simulink model "linearPathDomainPlnt_th"  (R2018a)
settings: Solver=FixedStepAuto  StartTime=0.0  StopTime=simulationDuration_s  FixedStep=simulationTimeStep_s  RelTol=1e-3
libraries: linearPathDomainPlnt_cl x1
settings Model: Creator=mcobb  LastModifiedBy=mcobb

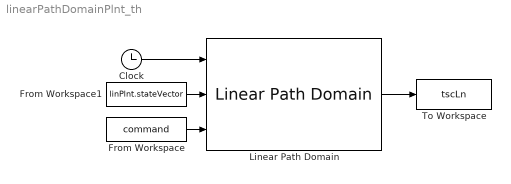
== system linearPathDomainPlnt_th ==
  Clock : Clock
  From Workspace : FromWorkspace  VariableName=command  SampleTime=0
  From Workspace1 : FromWorkspace  VariableName=linPlnt.stateVector  SampleTime=0
  Linear Path Domain : linearPathDomainPlnt_cl/Linear Path Domain  VariantControl=VSS_LINEARPATHDOMAIN_PLNT
  To Workspace : ToWorkspace  VariableName=tscLn  SaveFormat=Timeseries  SampleTime=-1
  wires:
  Linear Path Domain/1 -> To Workspace/1
  Clock/1 -> Linear Path Domain/1
  From Workspace/1 -> Linear Path Domain/3
  From Workspace1/1 -> Linear Path Domain/2
